simulink model "lab1_nonlinear_tau"  (R2024a)
settings: Solver=VariableStepAuto  StartTime=0.0  StopTime=10.0  RelTol=1e-3
values from neighbouring files (symbols this model uses):
  Cm = 1.3    [constants.m]
  Cw = 3.15    [constants.m]
  J_motor = 7*10^(-6)    (= 7e-06)    [constants.m]
  L_anhor = 0.0015    [constants.m]
  L_coils = 0.013    [constants.m]
  R_anhor = 8    [constants.m]
settings Model: Creator=nicka  LastModifiedBy=nicka

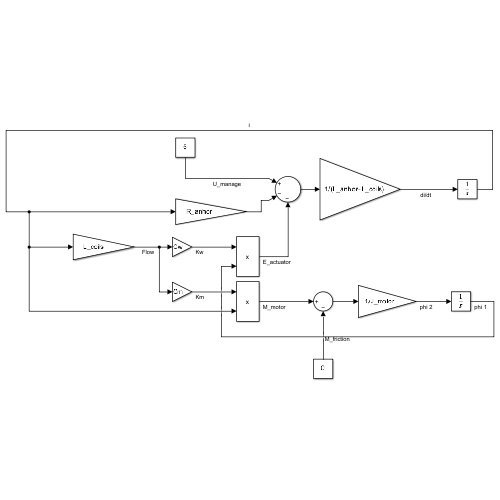
[thumbnail: Simulink's stored preview of the top-level diagram]
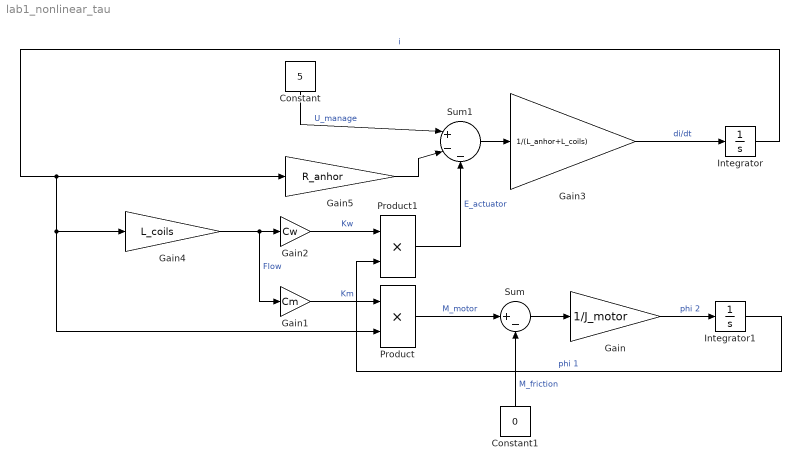
== system lab1_nonlinear_tau ==
  Constant : Constant  Value=5
  Constant1 : Constant  Value=0
  Gain : Gain  Gain=1/J_motor
  Gain1 : Gain  Gain=Cm
  Gain2 : Gain  Gain=Cw
  Gain3 : Gain  Gain=1/(L_anhor+L_coils)
  Gain4 : Gain  Gain=L_coils
  Gain5 : Gain  Gain=R_anhor
  Integrator : Integrator
  Integrator1 : Integrator
  Product : Product
  Product1 : Product
  Sum : Sum  Inputs=|+-
  Sum1 : Sum  Inputs=|+--
  wires:
  Constant/1 -> Sum1/1  "U_manage"
  Gain5/1 -> Sum1/2
  Gain4/1 -> Gain1/1, Gain2/1  "Flow"
  Gain2/1 -> Product1/1  "Kw"
  Product1/1 -> Sum1/3  "E_actuator"
  Sum1/1 -> Gain3/1
  Gain3/1 -> Integrator/1  "di/dt"
  Gain1/1 -> Product/1  "Km"
  Integrator/1 -> Product/2, Gain4/1, Gain5/1  "i"
  Product/1 -> Sum/1  "M_motor"
  Constant1/1 -> Sum/2  "M_friction"
  Sum/1 -> Gain/1
  Gain/1 -> Integrator1/1  "phi 2"
  Integrator1/1 -> Product1/2  "phi 1"
